simulink model "test_triggered_counter"  (Simulink 6.2)
settings: Solver=ode45  StartTime=0.0  StopTime=50  RelTol=1e-3
libraries: xbsIndex_r3 x4, simulink x1, newfft_library x1
settings Model: LastModifiedBy=mdexter
settings DebuggingCC: SolverPrmCheckMsg=warning

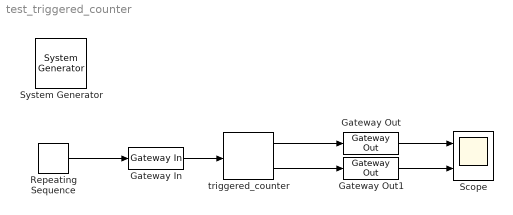
== system test_triggered_counter ==
  " System Generator" : xbsIndex_r3/ System Generator  Tag=genX  xilinxfamily=Virtex2P  part=xc2vp50  speed=-7  package=ff1152  synthesis_tool=XST  directory=./ibob_ata_ddc_8_sr/sysgen  testbench=off  simulink_period=1  sysclk_period=4.7684  incr_netlist=off  trim_vbits=Everywhere in SubSystem  dbl_ovrd=According to Block Masks  core_generation=According to Block Masks  run_coregen=off  deprecated_control=off  eval_field=0
      settings: AttributesFormatString=System\nGenerator
  Gateway In : xbsIndex_r3/Gateway In  arith_type=Boolean  n_bits=8  bin_pt=6  quantization=Truncate  overflow=Wrap  period=1  timing_constraint=None  locs_specified=off  LOCs={}  needs_fixed_name=off  dbl_ovrd=off  show_param=off
      settings: xl_area=[0, 0, 0, 0, 0, 0, 0]
  Gateway Out : xbsIndex_r3/Gateway Out  output_type=Double  nbits=8  bin_pt=6  arith_type=Boolean  quantization=Truncate  overflow=Wrap  hdl_port=on  timing_constraint=None  locs_specified=off  LOCs={}  needs_fixed_name=off  show_param=off
      settings: xl_area=[0, 0, 0, 0, 0, 0, 0]
  Gateway Out1 : xbsIndex_r3/Gateway Out  output_type=Double  nbits=8  bin_pt=6  arith_type=Boolean  quantization=Truncate  overflow=Wrap  hdl_port=on  timing_constraint=None  locs_specified=off  LOCs={}  needs_fixed_name=off  show_param=off
      settings: xl_area=[0, 0, 0, 0, 0, 0, 0]
  Repeating Sequence : simulink/Sources/Repeating Sequence  rep_seq_t=[0:32]  rep_seq_y=[zeros(1,22),1,zeros(1,10)]
  Scope : Scope  NumInputPorts=2
      settings: YMin=-5~-5  YMax=5~5
  triggered_counter : newfft_library/Utility/triggered_counter  len=8
  wires:
  Repeating Sequence/1 -> Gateway In/1
  Gateway Out/1 -> Scope/1
  Gateway Out1/1 -> Scope/2
  triggered_counter/1 -> Gateway Out/1
  Gateway In/1 -> triggered_counter/1
  triggered_counter/2 -> Gateway Out1/1
